simulink model "tst_bus_complex_incomplete"  (Simulink 8.0)
settings: Solver=ode45  StartTime=0.0  StopTime=10.0  RelTol=1e-3
settings Model: Creator=Marci  LastModifiedBy=massif

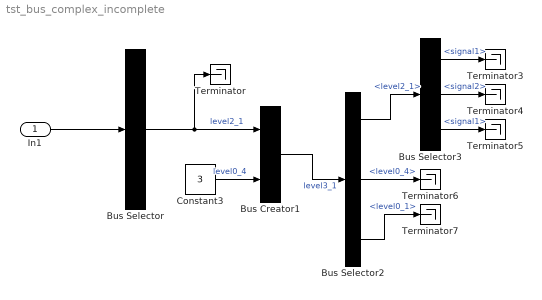
== system tst_bus_complex_incomplete ==
  In1 : Inport
  Bus Creator1 : BusCreator  Inputs=2
  Bus Selector : BusSelector  OutputSignals=level0_1,level0_2  OutputAsBus=on
  Bus Selector2 : BusSelector  OutputSignals=level2_1,level0_4,level2_1.level0_1
  Bus Selector3 : BusSelector  OutputSignals=signal1,signal2,signal1
  Constant3 : Constant  Value=3
  Terminator{,3..7} (6 alike) : Terminator
  wires:
  In1/1 -> Bus Selector/1
  Bus Selector/1 -> Terminator/1, Bus Creator1/1  "level2_1"
  Bus Creator1/1 -> Bus Selector2/1  "level3_1"
  Constant3/1 -> Bus Creator1/2  "level0_4"
  Bus Selector2/1 -> Bus Selector3/1  "<level2_1>"
  Bus Selector2/2 -> Terminator6/1  "<level0_4>"
  Bus Selector3/1 -> Terminator3/1  "<signal1>"
  Bus Selector3/2 -> Terminator4/1  "<signal2>"
  Bus Selector3/3 -> Terminator5/1  "<signal1>"
  Bus Selector2/3 -> Terminator7/1  "<level0_1>"
